simulink model "ArmSim"  (R2014a)
settings: Solver=FixedStepDiscrete  SolverMode=SingleTasking  StartTime=0.0  StopTime=100  FixedStep=dt  RelTol=1e-3
values from neighbouring files (symbols this model uses):
  dt = 0.01    [ballToss.m]
  dtheta1_throw_traj = [0, diff(theta1_throw_traj)/dt]    [ballToss.m]
  dtheta2_throw_traj = [0, diff(theta2_throw_traj)/dt]    [ballToss.m]
  theta1_throw_traj = [0 0 0 1.3 1.3 1.3 1.3 1.3 1.3 1.3]    [ballToss.m]
  theta2_throw_traj = [0 0 0 1 1 1 1 1 1 1]    [ballToss.m]
libraries: legonxtlib x4, cstblocks x2
settings Model: SimulationMode=external  ExtModeTrigDuration=2  Creator=syt  LastModifiedBy=yutongfeng
settings OptimizationCC: OptimizeModelRefInitCode=on  LifeSpan=1
settings DebuggingCC: UnderspecifiedInitializationDetection=Classic  SolverPrmCheckMsg=none
settings HardwareCC: ProdLargestAtomicInteger=Long  ProdLargestAtomicFloat=Float  ProdEndianess=LittleEndian  ProdHWDeviceType=ARM Compatible->ARM 7
settings RTWCC: SystemTargetFile=realtime.tlc  GenerateMakefile=off  TemplateMakefile=realtime.tmf  Description=Run on Target Hardware  RTWVerbose=off  ProcessScript=realtime_make_rtw_hook
settings STFCustomTargetCC: TargetLibSuffix=.a  GenerateSampleERTMain=on  ConcurrentExecutionCompliant=off  GeneratePreprocessorConditionals=Use local settings  ERTCustomFileBanners=on  SupportNonInlinedSFcns=off  SupportVariableSizeSignals=on  MATLABClassNameForMDSCustomization=Simulink.SoftwareTarget.ERTCustomization  GRTInterface=off  SystemTargetFile=realtime.tlc
settings ERTTargetCC: CombineOutputUpdateFcns=off  SupportContinuousTime=on  SupportVariableSizeSignals=on  ExtMode=on  ExtModeTransport=2  ExtModeMexFile=ext_serial_win32_comm_no_acks_rtt  ExtModeMexArgs=0 114 9600 30  ERTSrcFileBannerTemplate=realtime_code_template.cgt  ERTHdrFileBannerTemplate=realtime_code_template.cgt  ERTDataSrcFileTemplate=realtime_code_template.cgt  ERTDataHdrFileTemplate=realtime_code_template.cgt  ERTCustomFileTemplate=realtime_file_process.tlc

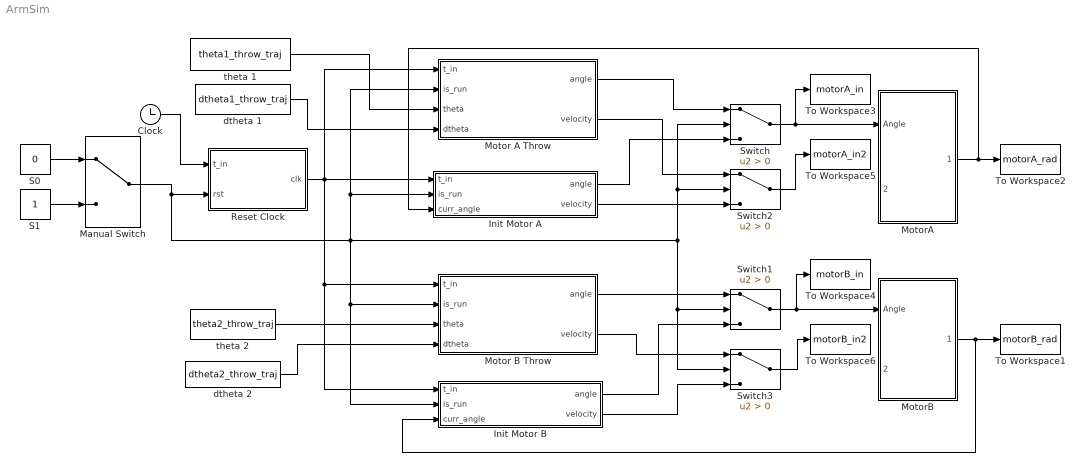
== system ArmSim ==
  Clock : Clock
  Init Motor A : MATLAB Function  TreatAsAtomicUnit=on
  Init Motor B : MATLAB Function  TreatAsAtomicUnit=on
  Manual Switch : ManualSwitch
  Motor A Throw : MATLAB Function  TreatAsAtomicUnit=on
  Motor B Throw : MATLAB Function  TreatAsAtomicUnit=on
  MotorA : Subsystem
  MotorB : Subsystem
  Reset Clock : MATLAB Function  TreatAsAtomicUnit=on
  S0 : Constant  Value=0
  S1 : Constant
  Switch{,1..3} (4 alike) : Switch  Criteria=u2 > Threshold
  To Workspace1 : ToWorkspace  VariableName=motorB_rad  SaveFormat=Structure With Time  SampleTime=-1
  To Workspace2 : ToWorkspace  VariableName=motorA_rad  SaveFormat=Structure With Time  SampleTime=-1
  To Workspace3 : ToWorkspace  VariableName=motorA_in  SaveFormat=Structure With Time  SampleTime=-1
  To Workspace4 : ToWorkspace  VariableName=motorB_in  SaveFormat=Structure With Time  SampleTime=-1
  To Workspace5 : ToWorkspace  VariableName=motorA_in2  SaveFormat=Structure With Time  SampleTime=-1
  To Workspace6 : ToWorkspace  VariableName=motorB_in2  SaveFormat=Structure With Time  SampleTime=-1
  dtheta 1 : Constant  Value=dtheta1_throw_traj
  dtheta 2 : Constant  Value=dtheta2_throw_traj
  theta 1 : Constant  Value=theta1_throw_traj
  theta 2 : Constant  Value=theta2_throw_traj
  wires:
  S0/1 -> Manual Switch/1
  S1/1 -> Manual Switch/2
  Clock/1 -> Reset Clock/1(t_in)
  Manual Switch/1 -> Init Motor B/2(is_run), Motor B Throw/2(is_run), Motor A Throw/2(is_run), Init Motor A/2(is_run), Switch3/2, Switch1/2, Switch/2, Switch2/2, Reset Clock/2(rst)
  Switch/1 -> MotorA/1(Angle), To Workspace3/1
  Switch1/1 -> MotorB/1(Angle), To Workspace4/1
  Motor A Throw/1(angle) -> Switch/1
  Reset Clock/1(clk) -> Init Motor B/1(t_in), Motor B Throw/1(t_in), Init Motor A/1(t_in), Motor A Throw/1(t_in)
  Motor A Throw/2(velocity) -> Switch2/1
  MotorA/1(actual_angle) -> Init Motor A/3(curr_angle), To Workspace2/1
  MotorB/1(actual angle) -> Init Motor B/3(curr_angle), To Workspace1/1
  dtheta 1/1 -> Motor A Throw/4(dtheta)
  theta 1/1 -> Motor A Throw/3(theta)
  Switch2/1 -> To Workspace5/1
  Init Motor A/2(velocity) -> Switch2/3
  Init Motor A/1(angle) -> Switch/3
  theta 2/1 -> Motor B Throw/3(theta)
  dtheta 2/1 -> Motor B Throw/4(dtheta)
  Motor B Throw/1(angle) -> Switch1/1
  Motor B Throw/2(velocity) -> Switch3/1
  Init Motor B/1(angle) -> Switch1/3
  Init Motor B/2(velocity) -> Switch3/3
  Switch3/1 -> To Workspace6/1

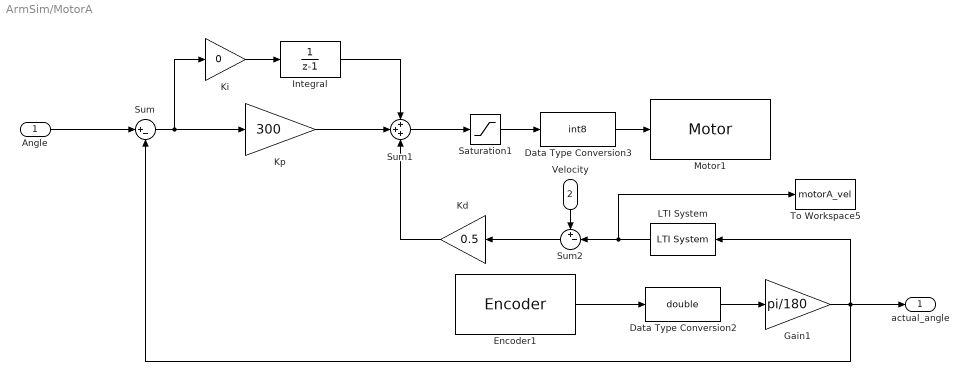
== system ArmSim/MotorA ==
  Angle : Inport
  Velocity : Inport  Port=2
  Data Type Conversion2 : DataTypeConversion  OutDataTypeStr=double
  Data Type Conversion3 : DataTypeConversion  OutDataTypeStr=int8
  Encoder1 : legonxtlib/Encoder  portNumber=A  opMode=No reset  sampleTime=dt
  Gain1 : Gain  Gain=pi/180
  Integral : DiscreteTransferFcn  Denominator=[1 -1]  SampleTime=dt
  Kd : Gain  Gain=0.5
  Ki : Gain  Gain=0
  Kp : Gain  Gain=300
  LTI System : cstblocks/LTI System  sys=dttf  IC=[]
  Motor1 : legonxtlib/Motor  sportNumber=A  sstopAction=Brake
  Saturation1 : Saturate  UpperLimit=100  LowerLimit=-100
  Sum : Sum  Inputs=|+-
  Sum1 : Sum  Inputs=+++
  Sum2 : Sum  Inputs=+-|
  To Workspace5 : ToWorkspace  VariableName=motorA_vel  SaveFormat=Structure With Time  SampleTime=-1
  actual_angle : Outport
  wires:
  Encoder1/1 -> Data Type Conversion2/1
  Data Type Conversion2/1 -> Gain1/1
  Data Type Conversion3/1 -> Motor1/1
  Saturation1/1 -> Data Type Conversion3/1
  Angle/1 -> Sum/1
  Sum1/1 -> Saturation1/1
  LTI System/1 -> To Workspace5/1, Sum2/2
  Gain1/1 -> LTI System/1, actual_angle/1, Sum/2
  Velocity/1 -> Sum2/1
  Sum2/1 -> Kd/1
  Sum/1 -> Ki/1, Kp/1
  Ki/1 -> Integral/1
  Integral/1 -> Sum1/1
  Kp/1 -> Sum1/2
  Kd/1 -> Sum1/3

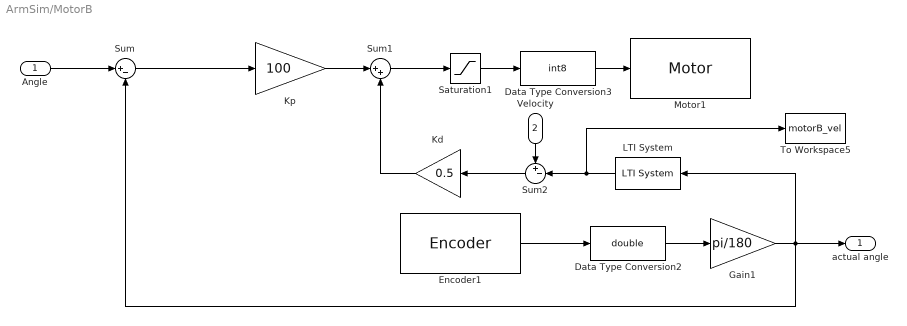
== system ArmSim/MotorB ==
  Angle : Inport
  Velocity : Inport  Port=2
  Data Type Conversion2 : DataTypeConversion  OutDataTypeStr=double
  Data Type Conversion3 : DataTypeConversion  OutDataTypeStr=int8
  Encoder1 : legonxtlib/Encoder  portNumber=B  opMode=No reset  sampleTime=dt
  Gain1 : Gain  Gain=pi/180
  Kd : Gain  Gain=0.5
  Kp : Gain  Gain=100
  LTI System : cstblocks/LTI System  sys=dttf  IC=[]
  Motor1 : legonxtlib/Motor  sportNumber=B  sstopAction=Brake
  Saturation1 : Saturate  UpperLimit=100  LowerLimit=-100
  Sum : Sum  Inputs=|+-
  Sum1 : Sum  Inputs=|++
  Sum2 : Sum  Inputs=+-|
  To Workspace5 : ToWorkspace  VariableName=motorB_vel  SaveFormat=Structure With Time  SampleTime=-1
  actual angle : Outport
  wires:
  Encoder1/1 -> Data Type Conversion2/1
  Data Type Conversion2/1 -> Gain1/1
  Gain1/1 -> LTI System/1, actual angle/1, Sum/2
  Data Type Conversion3/1 -> Motor1/1
  Saturation1/1 -> Data Type Conversion3/1
  Angle/1 -> Sum/1
  Sum/1 -> Kp/1
  Kp/1 -> Sum1/1
  Sum1/1 -> Saturation1/1
  LTI System/1 -> To Workspace5/1, Sum2/2
  Velocity/1 -> Sum2/1
  Sum2/1 -> Kd/1
  Kd/1 -> Sum1/2

== matlab function ArmSim/Motor A Throw ==
  data: angle output; t_in input; is_run input; theta input; dtheta input; velocity output
function [angle, velocity] = motor_throw(t_in, is_run, theta, dtheta)
persistent count t_curr
if isempty(count)
    count = 0;
end
if isempty(t_curr)
    t_curr = 0;
end

if is_run == 0
    count = 0;
    t_curr = 0;
    angle = 0;
    velocity = 0;
else
    if (t_in > t_curr) && (count < length(theta))
        count = count +1;
    end
    velocity = dtheta(count);
    angle = theta(count);   
    t_curr = t_in;
end

== matlab function ArmSim/Reset Clock ==
  data: t_in input; clk output; rst input
function clk = reset_clock(t_in, rst)
persistent t_off last_rst
if isempty(t_off)
    t_off = 0;
end
if isempty(last_rst)
    last_rst = 0;
end

if abs(rst -last_rst) ~= 0
    t_off = t_in;
end

clk = t_in -t_off;
last_rst = rst;

== matlab function ArmSim/Init Motor A ==
  data: t_in input; is_run input; angle output; velocity output; curr_angle input
function [angle, velocity] = back_motor(t_in, is_run, curr_angle)
Back_Time = 2;
persistent max_angle
if isempty(max_angle)
    max_angle = 0;
end

if is_run > 0
    max_angle = curr_angle;
    angle = 0;
    velocity = 0;
else
    back_ratio = 1-(t_in/Back_Time);
    if back_ratio > 0
        angle = max_angle*back_ratio;
        velocity = 0;
    else
        angle = 0;
        velocity = 0;
    end
end

== matlab function ArmSim/Motor B Throw ==
  data: angle output; t_in input; is_run input; theta input; dtheta input; velocity output
function [angle, velocity] = motor_throw(t_in, is_run, theta, dtheta)
persistent count t_curr
if isempty(count)
    count = 0;
end
if isempty(t_curr)
    t_curr = 0;
end

if is_run == 0
    count = 0;
    t_curr = 0;
    angle = 0;
    velocity = 0;
else
    if (t_in > t_curr) && (count < length(theta))
        count = count +1;
    end
    velocity = dtheta(count);
    angle = theta(count);   
    t_curr = t_in;
end

== matlab function ArmSim/Init Motor B ==
  data: t_in input; is_run input; angle output; velocity output; curr_angle input
function [angle, velocity] = back_motor(t_in, is_run, curr_angle)
Back_Time = 2;
persistent max_angle
if isempty(max_angle)
    max_angle = 0;
end

if is_run > 0
    max_angle = curr_angle;
    angle = 0;
    velocity = 0;
else
    back_ratio = 1-(t_in/Back_Time);
    if back_ratio > 0
        angle = max_angle*back_ratio;
        velocity = 0;
    else
        angle = 0;
        velocity = 0;
    end
end
